simulink model "practica13"  (R2015a)
settings: Solver=ode45  StartTime=0.0  StopTime=10  RelTol=1e-3
libraries: simulink x1
settings Model: Creator=Alumnos  LastModifiedBy=Alumnos

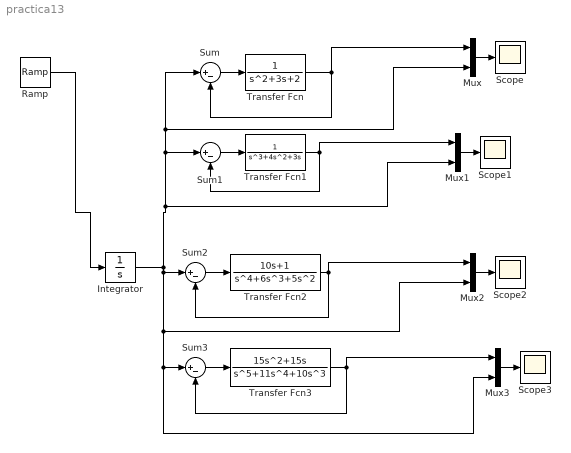
== system practica13 ==
  Integrator : Integrator
  Mux{,1..3} (4 alike) : Mux  Inputs=2
  Ramp : simulink/Sources/Ramp  slope=1  start=0  X0=0
  Scope{,1..3} (4 alike) : Scope
      Scope2 settings: SaveName=ScopeData2
      Scope3 settings: YMin=-1e+10  YMax=3.5e+10  SaveName=ScopeData3
  Sum{,1..3} (4 alike) : Sum  Inputs=|+-
  Transfer Fcn : TransferFcn  Denominator=[1 3 2]
  Transfer Fcn1 : TransferFcn  Denominator=[1 4 3 0]
  Transfer Fcn2 : TransferFcn  Numerator=[10 1]  Denominator=[1 6 5 0 0]
  Transfer Fcn3 : TransferFcn  Numerator=[15 15 0]  Denominator=[1 11 10 0 0 0]
  wires:
  Transfer Fcn/1 -> Sum/2, Mux/1
  Transfer Fcn1/1 -> Sum1/2, Mux1/1
  Sum/1 -> Transfer Fcn/1
  Sum1/1 -> Transfer Fcn1/1
  Sum2/1 -> Transfer Fcn2/1
  Sum3/1 -> Transfer Fcn3/1
  Mux/1 -> Scope/1
  Mux1/1 -> Scope1/1
  Transfer Fcn2/1 -> Sum2/2, Mux2/1
  Mux2/1 -> Scope2/1
  Transfer Fcn3/1 -> Sum3/2, Mux3/1
  Mux3/1 -> Scope3/1
  Ramp/1 -> Integrator/1
  Integrator/1 -> Mux1/2, Sum1/1, Mux/2, Sum/1, Mux2/2, Mux3/2, Sum3/1, Sum2/1
